simulink model "LabFabSim2022a__2_9_2023_AllAttacks_"  (R2022a)
settings: Solver=VariableStepAuto  StartTime=0.0  StopTime=5500000  RelTol=1e-3  EnableMultiTasking=on
model workspace (MAT data in the model file):
  JsonData : timetable (value not decoded)
  M : Simulink.Parameter (value not decoded)
  ROS_trigger = 0
  SL_ROS_VariableLengthArrays_MaxSizes : object (value not decoded)
undefined symbols (not defined in the file): DOS, DOSinitGen, DTP, DTPGen, DTPInitGen, EmptyLocFound, InitCobot, InitCobotReturn, InitializeSLD, InitLEGO, InitVGRproc2, m, MC, MCGen, MCInitGen, MO, MOGen, MOInitGen, n, NetScan, NetScanInitGen, Spying, SpyingInitGen, WS, WSGen, WSInitGen
libraries: sldelib x6
(part 2 of 4)

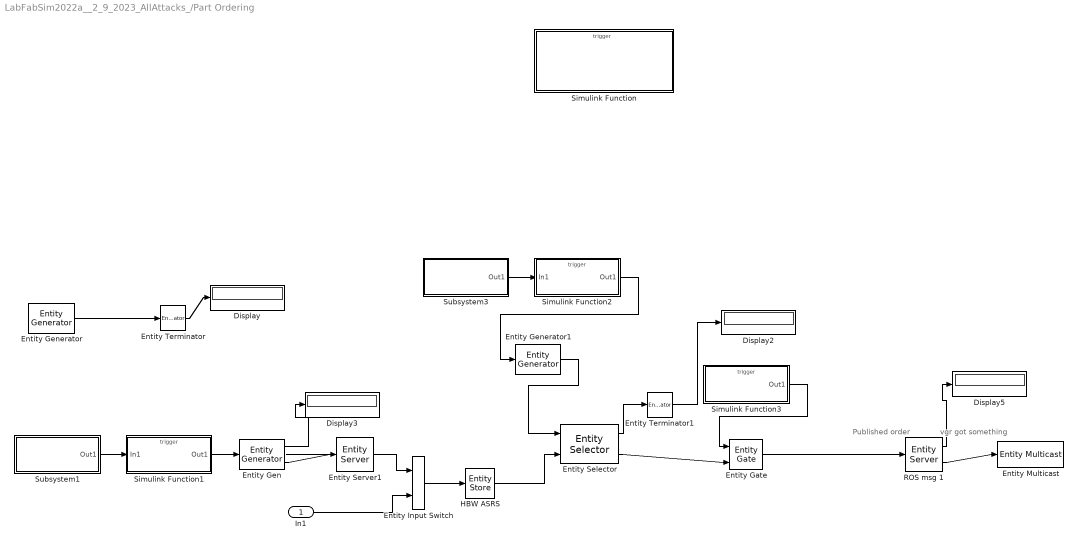
== system LabFabSim2022a__2_9_2023_AllAttacks_/Part Ordering ==
  note: vgr got something
  note: Published order
  In1 : Inport
  Display{,2..3,5} (4 alike) : Display
  Entity Input Switch : EntityInputSwitch  InputPortMessageModes=m,m  OutputPortMessageModes=m
  Entity Gate : EntityGate  InputPortMessageModes=m,m  OutputPortMessageModes=m  OperatingMode=Release gate  OpenGateAtSimulationStart=on
  "Entity Gen " : EntityGenerator  InputPortMessageModes=m  OutputPortMessageModes=n,m  GenerationMethod=Event-based  GenerateAction=|  AttributeName=PartID|ColorID|ServiceProcess|CurrentStep|CurrentRoute|HBW_ServiceTime|LEGO_ServiceTime|SLD_ServiceTime|HBW_Loc|TimeStampGen|TimeStampEnd|TimeStampStart|TotalTimeInSys|EntityRoutedTime|HBWstart_Time|VGRproc1_Time|MPS_Time|SLD_Time|VGRproc2_Time|Cobot2LEGO_Time|LEGO2Cobot_Time|VGRproc3_Time|HBWin_Time  AttributeInitialValue=1|1|zeros(1,11)|0|1|zeros(1)|zeros(1)|zeros(1)|zeros(1)|0|0|0|0|0|0|0|0|0|0|0|0|0|0  NumberEntitiesDeparted=on  EntityType=Structured  EntityTypeName=PartOrder
      | persistent next_id
      | if isempty(next_id)
      |     next_id = 1;
      |     %set seed for random number generation
      |     rng(12345);
      | end
      | 
      | %Assign ID attribute 
      | if next_id <= 9
      |     entity.PartID = next_id;
      |     next_id = next_id + 1
      | end
      | 
      | %Current Step Attribute Setup
      | persistent SEQId;
      | persistent idx2;
      | if isempty(SEQId)
      |     SEQId = 1:15;
      |     idx2 = 1;
      | end
      | if idx2 > numel(SEQId)
      |     idx2 = 1;
      |     entity.PartID = SEQId(idx2);
      | else
      |     entity.PartID = SEQId(idx2);
      | end
      | idx2 = idx2 + 1;
      | entity.CurrentStep=1;
      | 
      | %Randomly Set Order Color 
      | entity.HBW_Loc = randi(3)
      | switch(entity.HBW_Loc)
      |     case 1 
      |         entity.ColorID = 1;
      |         %entity.Color = "red";
      |         %red part ordered
      |     case 2
      |         entity.ColorID = 2;
      |         %entity.Color = "blue";
      |         %blue part ordered 
      |     case 3 
      |         entity.ColorID = 3;
      |         %entity.Color = "white";
      |         %white part ordered 
      | end
      | 
      | %Entity attribute based on color ID
      | if entity.ColorID == 1
      |     entity.ServiceProcess = [2 3 4 5 6 7 8 9 10 11 1];
      |     entity.HBW_ServiceTime = [5];
      |     entity.LEGO_ServiceTime = [4];
      |     entity.SLD_ServiceTime = [6];
      |     
      | else if entity.ColorID == 2
      |     entity.ServiceProcess = [2 3 4 5 6 7 8 9 10 11 1];
      |     entity.HBW_ServiceTime = [6];
      |     entity.LEGO_ServiceTime = [4];
      |     entity.SLD_ServiceTime = [7];
      |     
      | else if entity.ColorID == 3
      |     entity.ServiceProcess = [2 3 4 5 6 7 8 9 10 11 1];
      |     entity.HBW_ServiceTime = [5];
      |     entity.LEGO_ServiceTime = [6];
      |     entity.SLD_ServiceTime = [5];
      | end
      | end
      settings: InputPortMap=u0  OutputPortMap=o0,o3
  Entity Generator : EntityGenerator  OutputPortMessageModes=m  Period=inf  AttributeName=data  EntityType=Structured  EntityTypeName=InitOrders
  Entity Generator1 : EntityGenerator  InputPortMessageModes=m  OutputPortMessageModes=m  GenerationMethod=Event-based  GenerateAction=entity.PartID = randi(9);  AttributeName=PartID  AttributeInitialValue=zeros(1)  EntityType=Structured  EntityTypeName=Order
      settings: InputPortMap=u0
  Entity Multicast : EntityMulticast  Tag=Order  InputPortMessageModes=m  MulticastTag=Order
  Entity Selector : sldelib/Entity Selector  mNumberOfStreams=1  mKeyEntityAttributeName={'PartID'}  mEntityAttributeName={'PartID'}  mMatchingNumberSource=Dialog  mNumberOfMatches=1  mNumberOfMatchesAttribute=Name  mNumEntitiesDepOpt=off  mNumEntitiesInBlockOpt=off  mNumEntitiesExtractedOpt=off
      settings: SourceProductBaseCode=SE
  Entity Server1 : EntityServer  InputPortMessageModes=m  OutputPortMessageModes=m  Capacity=1  ServiceTimeValue=0  EntryAction=entity.TimeStampGen = TimeStamp();
  Entity Terminator : EntityTerminator  InputPortMessageModes=m  EntryAction=|  NumberEntitiesArrived=on
      | EntityGen();
      | EntityGen();
      | EntityGen();
      | EntityGen();
      | EntityGen();
      | EntityGen();
      | EntityGen();
      | EntityGen();
      | EntityGen();
      | 
      | %Initially set attack Routers to closed state
      | DOS_Router(2);
      | NetScan_Router(2);
      | Spying_Router(2);
      | DTP_Router(2);
      | MO_Router(2);
      | WS_Router(2);
      | MC_Router(2);
      | 
      | 
      | % coder.extrinsic("disp");
      | 
      | % a = [1, 1; 
      | %     2, 1; 
      | %     3, 1; 
      | %     4, 1; 
      | %     5, 1; 
      | %     6, 1; 
      | %     7, 1; 
      | %     8, 1; 
      | %     9, 1];
      | % b = [datetime('now'); datetime('now'); datetime('now'); datetime('now'); datetime('now'); datetime('now'); datetime('now'); datetime('now'); datetime('now')];
      | % JsonDataSTART= array2timetable(a, 'VariableNames', {'PartID', 'State'}, 'RowTimes', b);
      | % disp(JsonDataSTART)
      settings: OutputPortMap=o0
  Entity Terminator1 : EntityTerminator  InputPortMessageModes=m  NumberEntitiesArrived=on
      settings: OutputPortMap=o0
  HBW ASRS : EntityStore  InputPortMessageModes=m  OutputPortMessageModes=m  Capacity=9  EntryAction=|  ExitAction=|
      EntryAction=|
      | OrderGen();
      | 
      | % % coder.extrinsic("disp");
      | % % 
      | % % 
      | % %%% JSON UPDATE on part entry %%
      | % % if entity.PartID == 1
      | % %     JsonData.PartID(1) = 1;
      | % %     JsonData.Time(1) = datetime('now');
      | % %     
      | % % elseif entity.PartID == 2
      | % %     JsonData.PartID(2) = 2;
      | % %     JsonData.Time(2) = datetime('now');
      | % %     
      | % % elseif entity.PartID == 3
      | % %     JsonData.PartID(3) = 3;
      | % %     JsonData.Time(3) = datetime('now');
      | % %     
      | % % elseif entity.PartID == 4
      | % %     JsonData.PartID(4) = 4;
      | % %     JsonData.Time(4) = datetime('now');
      | % %     
      | % % elseif entity.PartID == 5
      | % %     JsonData.PartID(5) = 5;
      | % %     JsonData.Time(5) = datetime('now');
      | % %     
      | % % elseif entity.PartID == 6
      | % %     JsonData.PartID(6) = 6;
      | % %     JsonData.Time(6) = datetime('now');
      | % %     
      | % % elseif entity.PartID == 7
      | % %     JsonData.PartID(7) = 7;
      | % %     JsonData.Time(7) = datetime('now');
      | % %     
      | % % elseif entity.PartID == 8
      | % %     JsonData.PartID(8) = 8;
      | % %     JsonData.Time(8) = datetime('now');
      | % %     
      | % % elseif entity.PartID == 9
      | % %     JsonData.PartID(9) = 9;
      | % %     JsonData.Time(9) = datetime('now');
      | % % end
      | % % 
      | % % disp(JsonData)
      ExitAction=|
      | % % % %UpdateArrayOUT();
      | % coder.extrinsic("disp");
      | % a = [1, 1; 2, 1; 3, 1; 4, 1; 5, 1; 6, 1; 7, 1; 8, 1; 9, 1];
      | % % b = [datetime('now')];
      | % 
      | % %% JSON UPDATE on part exit %%
      | % if entity.PartID == 1
      | %     a(1,2) = 0;
      | %     %b(1) = datetime('now');
      | %     %disp(a)
      | %     
      | % elseif entity.PartID == 2
      | %     a(2,2) = 0;
      | %     %b(2) = datetime('now');
      | %     %disp(a)
      | %     
      | % elseif entity.PartID == 3
      | %     a(3,2) = 0;
      | %     %b(3) = datetime('now');
      | %     %disp(a)
      | %     
      | % elseif entity.PartID == 4
      | %     a(4,2) = 0;
      | %     %b(4) = datetime('now');
      | %     %disp(a)
      | %     
      | % elseif entity.PartID == 5
      | %     a(5,2) = 0;
      | %     %b(5) = datetime('now');
      | %     %disp(a)
      | %     
      | % elseif entity.PartID == 6
      | %     a(6,2) = 0;
      | %     %b(6) = datetime('now');
      | %     %disp(a)
      | %     
      | % elseif entity.PartID == 7
      | %     a(7,2) = 0;
      | %     %b(7) = datetime('now');
      | %     %disp(a)
      | %     
      | % elseif entity.PartID == 8
      | %     a(8,2) = 0;
      | %     %b(8) = datetime('now');
      | %     %disp(a)
      | %     
      | % elseif entity.PartID == 9
      | %     a(9,2) = 0;
      | %     %b(9) = datetime('now');
      | %     %disp(a)
      | % end
      | % 
      | % disp('____')
      | % JsonDataUPDATE= array2table(a, 'VariableNames', {'PartID', 'State'});
      | % disp(JsonDataUPDATE)
      settings: OutputPortMap=o4
  ROS msg 1 : EntityServer  InputPortMessageModes=m  OutputPortMessageModes=n,m  Capacity=1  ServiceTimeValue=0.07  EntryAction=|  ExitAction=|  NumberEntitiesDeparted=on
      EntryAction=|
      | entity.TimeStampStart = TimeStamp();
      | 
      | sourceID(3); %main
      | sourceAddress(6); %/order
      | sourceType(4); %order
      | sourceLocation(3); %SCADA system
      | destinationServiceAddress(1); %/hbw_node
      | destinationServiceType(4); %order
      | destinationServiceLocation(1); %Fischertechnik
      | accessedNodeAddress(7); 
      | accessedNodeType(1); %String
      | operation(3); %notify-callback
      | value(41); %Published order
      | Normality(1); %normal
      ExitAction=|
      | sourceID(3); %main
      | sourceAddress(6); %/order
      | sourceType(4); %order
      | sourceLocation(3); %SCADA system
      | destinationServiceAddress(2); %/vgr_node
      | destinationServiceType(4); %order
      | destinationServiceLocation(1); %Fischertechnik
      | accessedNodeAddress(3); 
      | accessedNodeType(1); %String
      | operation(3); %notify-callback
      | value(28); %Published order
      | Normality(1); %normal
      settings: OutputPortMap=o0,o9
  Simulink Function : Subsystem  TreatAsAtomicUnit=on
  Simulink Function1 : Subsystem  TreatAsAtomicUnit=on
  Simulink Function2 : Subsystem  TreatAsAtomicUnit=on
  Simulink Function3 : Subsystem  TreatAsAtomicUnit=on
  Subsystem1 : Subsystem
  Subsystem3 : Subsystem
  wires:
  Entity Terminator/1 -> Display/1
  Subsystem1/1(Out1) -> Simulink Function1/1(In1)
  Simulink Function1/1(Out1) -> "Entity Gen "/1
  HBW ASRS/1 -> Entity Selector/2
  Simulink Function3/1(Out1) -> Entity Gate/1
  ROS msg 1/2 -> Entity Multicast/1
  ROS msg 1/1 -> Display5/1
  "Entity Gen "/1 -> Display3/1
  "Entity Gen "/2 -> Entity Server1/1
  In1/1 -> Entity Input Switch/2
  Entity Selector/1 -> Entity Terminator1/1
  Entity Generator1/1 -> Entity Selector/1
  Subsystem3/1(Out1) -> Simulink Function2/1(In1)
  Simulink Function2/1(Out1) -> Entity Generator1/1
  Entity Terminator1/1 -> Display2/1
  Entity Generator/1 -> Entity Terminator/1
  Entity Input Switch/1 -> HBW ASRS/1
  Entity Server1/1 -> Entity Input Switch/1
  Entity Selector/2 -> Entity Gate/2
  Entity Gate/1 -> ROS msg 1/1

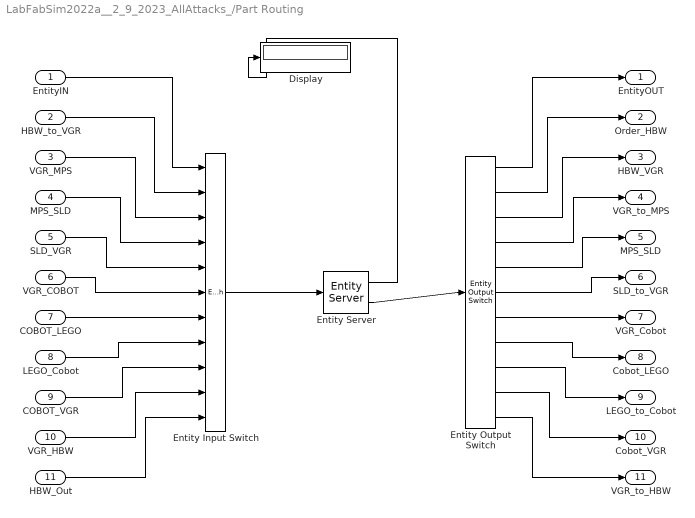
== system LabFabSim2022a__2_9_2023_AllAttacks_/Part Routing ==
  EntityIN : Inport
  HBW_to_VGR : Inport  Port=2
  VGR_MPS : Inport  Port=3
  MPS_SLD : Inport  Port=4
  SLD_VGR : Inport  Port=5
  VGR_COBOT : Inport  Port=6
  COBOT_LEGO : Inport  Port=7
  LEGO_Cobot : Inport  Port=8
  COBOT_VGR : Inport  Port=9
  VGR_HBW : Inport  Port=10
  HBW_Out : Inport  Port=11
  Display : Display
  Entity Input Switch : EntityInputSwitch  InputPortMessageModes=m,m,m,m,m,m,m,m,m,m,m  OutputPortMessageModes=m  NumberInputPorts=11
      settings: InputPortMap=u1,u2,u3,u4,u5,u6,u7,u8,u9,u10,u11
  Entity Output Switch : EntityOutputSwitch  InputPortMessageModes=m  OutputPortMessageModes=m,m,m,m,m,m,m,m,m,m,m  NumberOutputPorts=11  SwitchingCriterion=From attribute  SwitchAttributeName=CurrentRoute
      settings: OutputPortMap=o0,o1,o2,o3,o4,o5,o6,o7,o8,o9,o10
  Entity Server : EntityServer  InputPortMessageModes=m  OutputPortMessageModes=n,m  Capacity=1  ServiceTimeValue=0  EntryAction=|  NumberEntitiesDeparted=on
      | entity.CurrentRoute = entity.ServiceProcess(entity.CurrentStep);
      | entity.CurrentStep = entity.CurrentStep + 1;
      | entity.EntityRoutedTime = TimeStamp();
      settings: OutputPortMap=o0,o9
  EntityOUT : Outport
  Order_HBW : Outport  Port=2
  "HBW_VGR " : Outport  Port=3
  VGR_to_MPS : Outport  Port=4
  "MPS_SLD " : Outport  Port=5
  SLD_to_VGR : Outport  Port=6
  VGR_Cobot : Outport  Port=7
  Cobot_LEGO : Outport  Port=8
  LEGO_to_Cobot : Outport  Port=9
  Cobot_VGR : Outport  Port=10
  VGR_to_HBW : Outport  Port=11
  wires:
  EntityIN/1 -> Entity Input Switch/1
  HBW_to_VGR/1 -> Entity Input Switch/2
  VGR_MPS/1 -> Entity Input Switch/3
  MPS_SLD/1 -> Entity Input Switch/4
  SLD_VGR/1 -> Entity Input Switch/5
  VGR_COBOT/1 -> Entity Input Switch/6
  COBOT_LEGO/1 -> Entity Input Switch/7
  Entity Input Switch/1 -> Entity Server/1
  Entity Server/2 -> Entity Output Switch/1
  Entity Output Switch/1 -> EntityOUT/1
  Entity Output Switch/2 -> Order_HBW/1
  Entity Output Switch/3 -> "HBW_VGR "/1
  Entity Output Switch/4 -> VGR_to_MPS/1
  Entity Output Switch/5 -> "MPS_SLD "/1
  Entity Output Switch/6 -> SLD_to_VGR/1
  Entity Output Switch/7 -> VGR_Cobot/1
  Entity Server/1 -> Display/1
  Entity Output Switch/8 -> Cobot_LEGO/1
  Entity Output Switch/9 -> LEGO_to_Cobot/1
  Entity Output Switch/10 -> Cobot_VGR/1
  Entity Output Switch/11 -> VGR_to_HBW/1
  LEGO_Cobot/1 -> Entity Input Switch/8
  COBOT_VGR/1 -> Entity Input Switch/9
  VGR_HBW/1 -> Entity Input Switch/10
  HBW_Out/1 -> Entity Input Switch/11

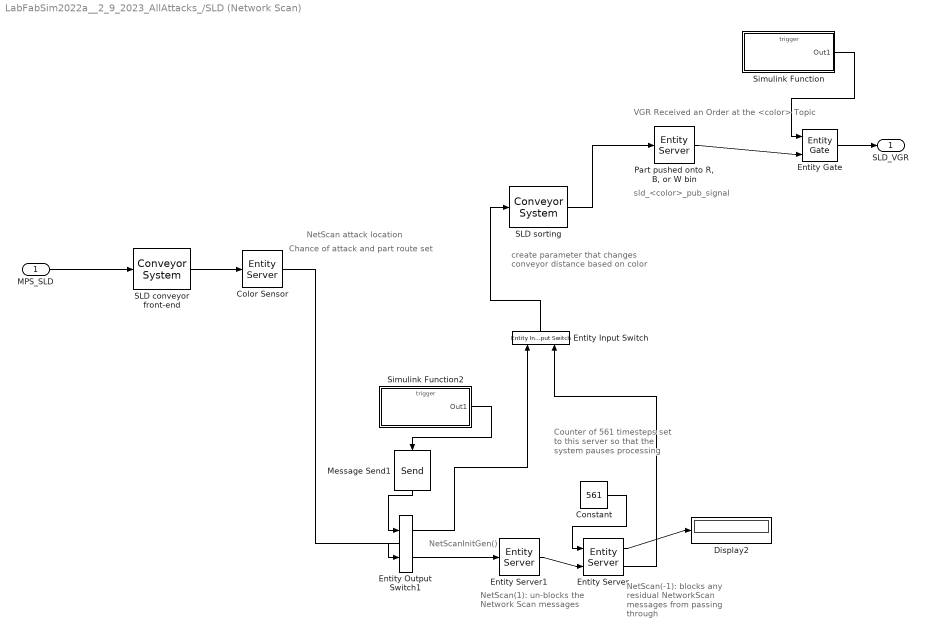
== system LabFabSim2022a__2_9_2023_AllAttacks_/SLD (Network Scan) ==
  note: VGR Received an Order at the <color> Topic
  note: sld_<color>_pub_signal
  note: create parameter that changes
      | conveyor distance based on color
  note: NetScanInitGen()
  note: NetScan(1):
      | un-blocks the Network Scan messages
  note: NetScan(-1):
      | blocks any residual NetworkScan messages from passing through
  note: Counter of 561 timesteps set to this server so that the system pauses processing
  note: Chance of attack and part route set
  note: NetScan attack location
  MPS_SLD : Inport
  Color Sensor : EntityServer  InputPortMessageModes=m  OutputPortMessageModes=m  Capacity=1  ExitAction=|
      | chanceNetScan = rand(1,1)
      | if chanceNetScan < 1.0
      |     %Attack Happening!
      |     NetScan_Router(1);
      | 
      | else
      |     %Normal Behavior
      |     NetScan(-1);
      |     NetScan_Router(2);
      | end
  Constant : Constant  Value=561
  Display2 : Display
  Entity Input Switch : EntityInputSwitch  InputPortMessageModes=m,m  OutputPortMessageModes=m
  Entity Output Switch1 : EntityOutputSwitch  InputPortMessageModes=m,m  OutputPortMessageModes=m,m  SwitchingCriterion=From control port  SwitchAttributeName=Attribute1
      settings: InputPortMap=u0,u1
  Entity Gate : EntityGate  InputPortMessageModes=m,m  OutputPortMessageModes=m  OperatingMode=Release gate
  Entity Server : EntityServer  InputPortMessageModes=n,m  OutputPortMessageModes=n,m  Capacity=1  ServiceTimeSource=Signal port  ExitAction=NetScan(-1);  NumberEntitiesDeparted=on
      settings: InputPortMap=u0,u2  OutputPortMap=o0,o9
  Entity Server1 : EntityServer  InputPortMessageModes=m  OutputPortMessageModes=m  Capacity=1  EntryAction=NetScanInitGen();  ServiceCompleteAction=NetScan(1);
  Message Send1 : Send  OutputPortMessageModes=m
  "Part pushed onto R, B, or W bin" : EntityServer  InputPortMessageModes=m  OutputPortMessageModes=m  Capacity=1  ServiceTimeSource=Attribute  ServiceTimeAttributeName=SLD_ServiceTime  EntryAction=InitVGRproc2();  ExitAction=|
      | sourceID(4); %sld
      | sourceAddress(7); %/vgr_node
      | sourceType(1); %motion sensor
      | sourceLocation(1); %Fischertechnik
      | destinationServiceAddress(2); %/vgr_node
      | destinationServiceType(5); %next task
      | destinationServiceLocation(1); %Fischertechnik
      | accessedNodeAddress(3); 
      | accessedNodeType(2); %String
      | operation(3); %notify-callback
      | Normality(1); %normal
      | 
      | if entity.ColorID == 1
      |     value(19); %VGR Received an Order at the RED Topic
      | else if entity.ColorID == 2
      |     value(18); %VGR Received an Order at the BLUE Topic
      | else    
      |     value(20); %VGR Received an Order at the WHITE Topic
      | end
  SLD conveyor front-end : sldelib/Conveyor System  mConveyorLength=100  mConveyorSpeedSource=Dialog  mConveyorSpeed=1000  mInitialConveyorSpeed=1000  mMinDisBetEntity=0  mEntityLengthSource=Dialog  mEntityLength=1  mEntityLengthAttrName=Length  mOutputBlockedOpt=Accumulate  mErrorUponFullOpt=on  mNumEntitiesDepOpt=off  mNumEntitiesInBlockOpt=off  mEntityPendingOpt=off  mNumExtractedFromBlockOpt=off  mConveyorSpeedOpt=off
      settings: SourceProductBaseCode=SE
  SLD sorting : sldelib/Conveyor System  mConveyorLength=100  mConveyorSpeedSource=Dialog  mConveyorSpeed=1000  mInitialConveyorSpeed=1000  mMinDisBetEntity=0  mEntityLengthSource=Dialog  mEntityLength=1  mEntityLengthAttrName=Length  mOutputBlockedOpt=Accumulate  mErrorUponFullOpt=on  mNumEntitiesDepOpt=off  mNumEntitiesInBlockOpt=off  mEntityPendingOpt=off  mNumExtractedFromBlockOpt=off  mConveyorSpeedOpt=off
      settings: SourceProductBaseCode=SE
  Simulink Function : Subsystem  TreatAsAtomicUnit=on
  Simulink Function2 : Subsystem  TreatAsAtomicUnit=on
  SLD_VGR : Outport
  wires:
  MPS_SLD/1 -> SLD conveyor front-end/1
  SLD conveyor front-end/1 -> Color Sensor/1
  SLD sorting/1 -> "Part pushed onto R, B, or W bin"/1
  "Part pushed onto R, B, or W bin"/1 -> Entity Gate/2
  Entity Gate/1 -> SLD_VGR/1
  Simulink Function/1(Out1) -> Entity Gate/1
  Entity Server/1 -> Display2/1
  Entity Server1/1 -> Entity Server/2
  Entity Server/2 -> Entity Input Switch/2
  Color Sensor/1 -> Entity Output Switch1/2
  Entity Input Switch/1 -> SLD sorting/1
  Constant/1 -> Entity Server/1
  Message Send1/1 -> Entity Output Switch1/1
  Entity Output Switch1/2 -> Entity Server1/1
  Entity Output Switch1/1 -> Entity Input Switch/1
  Simulink Function2/1(Out1) -> Message Send1/1

== system LabFabSim2022a__2_9_2023_AllAttacks_/Spying ==
  note: Source: hbw --> Destination: (2,5)
  note: Entity Gate:
      | set to open when a positive signal value is passed into the control port. Closes when negative.
  note: Recieve signal from Chance-setting Server block for activation signal
  note: Service Time: 50 Timestep
  note: Generates a single entity that causes Spying attack (entity generator) to generate one entity
  note: Sets Spying_id up to 5 and resets to 1 for next Spying attack
  note: On Service Completion: Send a signal to data-logging SimFunctions
  note: Service Time: 110 Timestep
  note: Service Time: 75 Timestep
  note: Service Time: 95 Timestep
  note: Service Time: 150 Timestep
  Display : Display
  Entity Gate : EntityGate  InputPortMessageModes=m,m  OutputPortMessageModes=m
  Entity Generator : EntityGenerator  InputPortMessageModes=m  OutputPortMessageModes=m  GenerationMethod=Event-based  IntergenerationTimeAction=|  GenerateAction=|  AttributeName=Spying_id  EntityType=Structured  EntityTypeName=SpyingAttack
      IntergenerationTimeAction=|
      | chanceDOS = rand(1,1);
      | if chanceDOS < 0.3
      |     dt = 1
      GenerateAction=|
      | persistent next_id_Spying
      | 
      | if isempty(next_id_Spying)
      |     next_id_Spying = 1;
      |     %set seed for random number generation
      |     rng(12345);
      | end
      | 
      | entity.Spying_id = next_id_Spying
      | next_id_Spying = next_id_Spying + 1
      | 
      | if entity.Spying_id == 5
      |     next_id_Spying = 1
      settings: InputPortMap=u0
  Entity Server : EntityServer  InputPortMessageModes=m  OutputPortMessageModes=m  Capacity=1  ServiceTimeValue=50  ServiceCompleteAction=|
      | sourceID(1); %hbw
      | sourceAddress(1); %/hbw_node
      | sourceType(5); %next_task
      | sourceLocation(1); %Fischertechnik
      | destinationServiceAddress(2); %/vgr_node
      | destinationServiceType(1); %Motion Sensor
      | destinationServiceLocation(1); %Fischertechnik
      | accessedNodeAddress(3); 
      | accessedNodeType(2); %Boolean
      | operation(1); %read
      | value(44); %False
      | Normality(6); %anomalous(spying)
  Entity Server1 : EntityServer  InputPortMessageModes=m  OutputPortMessageModes=m  Capacity=1  ServiceTimeValue=110  ServiceCompleteAction=|
      | sourceID(1); %hbw
      | sourceAddress(1); %/hbw_node
      | sourceType(5); %next_task
      | sourceLocation(1); %Fischertechnik
      | destinationServiceAddress(5); %/lego_node
      | destinationServiceType(1); %Motion Sensor
      | destinationServiceLocation(2); %Expansion
      | accessedNodeAddress(5); 
      | accessedNodeType(2); %Boolean
      | operation(1); %read
      | value(44); %False
      | Normality(6); %anomalous(spying)
  Entity Server2 : EntityServer  InputPortMessageModes=m  OutputPortMessageModes=m  Capacity=1  ServiceTimeValue=75  ServiceCompleteAction=|
      | sourceID(1); %hbw
      | sourceAddress(1); %/hbw_node
      | sourceType(5); %next_task
      | sourceLocation(1); %Fischertechnik
      | destinationServiceAddress(2); %/vgr_node
      | destinationServiceType(1); %Motion Sensor
      | destinationServiceLocation(1); %Fischertechnik
      | accessedNodeAddress(3); 
      | accessedNodeType(2); %Boolean
      | operation(1); %read
      | value(44); %False
      | Normality(6); %anomalous(spying)
  Entity Server3 : EntityServer  InputPortMessageModes=m  OutputPortMessageModes=m  Capacity=1  ServiceTimeValue=95  ServiceCompleteAction=|
      | sourceID(1); %hbw
      | sourceAddress(1); %/hbw_node
      | sourceType(5); %next_task
      | sourceLocation(1); %Fischertechnik
      | destinationServiceAddress(5); %/lego_node
      | destinationServiceType(1); %Motion Sensor
      | destinationServiceLocation(2); %Expansion
      | accessedNodeAddress(5);  
      | accessedNodeType(2); %Boolean
      | operation(1); %read
      | value(44); %False
      | Normality(6); %anomalous(spying)
  Entity Server4 : EntityServer  InputPortMessageModes=m  OutputPortMessageModes=m  Capacity=1  ServiceTimeValue=150  ServiceCompleteAction=|
      | sourceID(1); %hbw
      | sourceAddress(1); %/hbw_node
      | sourceType(5); %next_task
      | sourceLocation(1); %Fischertechnik
      | destinationServiceAddress(5); %/lego_node
      | destinationServiceType(1); %Motion Sensor
      | destinationServiceLocation(2); %Expansion
      | accessedNodeAddress(5);  
      | accessedNodeType(2); %Boolean
      | operation(1); %read
      | value(44); %False
      | Normality(6); %anomalous(spying)
  Entity Store : EntityStore  InputPortMessageModes=m  OutputPortMessageModes=m  Capacity=6
      settings: OutputPortMap=o4
  Entity Terminator1 : EntityTerminator  InputPortMessageModes=m  NumberEntitiesArrived=on
      settings: OutputPortMap=o0
  InitSpying : Subsystem
  "Number of Entities Generated from main " : Display
  Simulink Function1 : Subsystem  TreatAsAtomicUnit=on
  Spying : Subsystem  TreatAsAtomicUnit=on
  Subsystem1 : Subsystem
  wires:
  Simulink Function1/1(Out1) -> Entity Generator/1
  Entity Terminator1/1 -> Display/1
  Entity Generator/1 -> Entity Store/1
  Entity Store/1 -> Entity Gate/2
  Entity Server/1 -> Entity Server1/1
  Spying/1(Out1) -> Entity Gate/1
  Subsystem1/1(Out1) -> Simulink Function1/1(In1)
  InitSpying/1(Out1) -> "Number of Entities Generated from main "/1
  Entity Server1/1 -> Entity Server2/1
  Entity Server2/1 -> Entity Server3/1
  Entity Server3/1 -> Entity Server4/1
  Entity Server4/1 -> Entity Terminator1/1
  Entity Gate/1 -> Entity Server/1

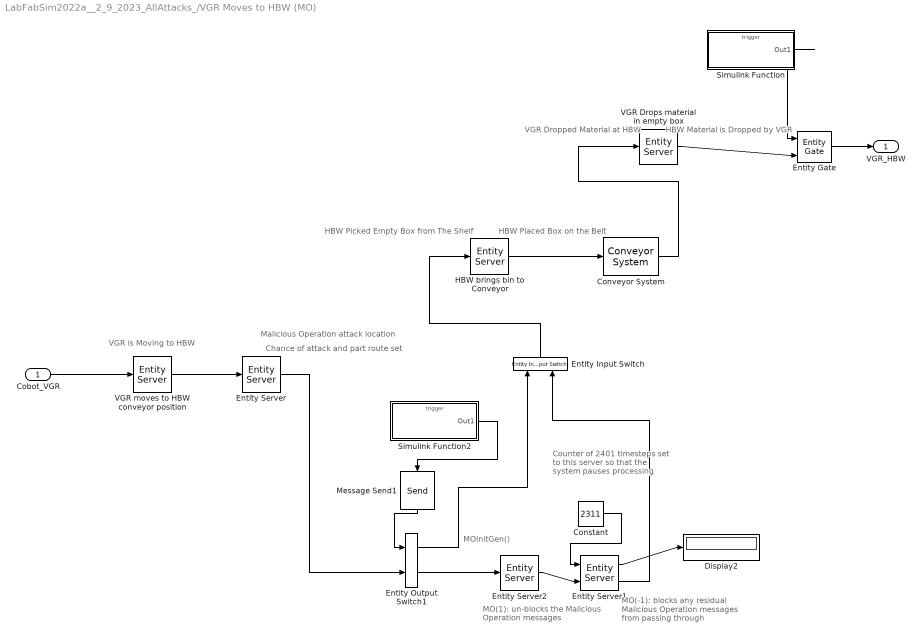
== system LabFabSim2022a__2_9_2023_AllAttacks_/VGR Moves to HBW (MO) ==
  note: HBW Material is Dropped by VGR
  note: VGR Dropped Material at HBW
  note: HBW Placed Box on the Belt
  note: HBW Picked Empty Box from The Shelf
  note: VGR is Moving to HBW
  note: MOInitGen()
  note: MO(-1):
      | blocks any residual Malicious Operation messages from passing through
  note: MO(1):
      | un-blocks the Malicious Operation messages
  note: Counter of 2401 timesteps set to this server so that the system pauses processing
  note: Malicious Operation attack location
  note: Chance of attack and part route set
  Cobot_VGR : Inport
  Constant : Constant  Value=2311
  Conveyor System : sldelib/Conveyor System  mConveyorLength=10  mConveyorSpeedSource=Dialog  mConveyorSpeed=1000  mInitialConveyorSpeed=1000  mMinDisBetEntity=0  mEntityLengthSource=Dialog  mEntityLength=1  mEntityLengthAttrName=Length  mOutputBlockedOpt=Accumulate  mErrorUponFullOpt=on  mNumEntitiesDepOpt=off  mNumEntitiesInBlockOpt=off  mEntityPendingOpt=off  mNumExtractedFromBlockOpt=off  mConveyorSpeedOpt=off
      settings: SourceProductBaseCode=SE
  Display2 : Display
  Entity Input Switch : EntityInputSwitch  InputPortMessageModes=m,m  OutputPortMessageModes=m
  Entity Output Switch1 : EntityOutputSwitch  InputPortMessageModes=m,m  OutputPortMessageModes=m,m  SwitchingCriterion=From control port  SwitchAttributeName=Attribute1
      settings: InputPortMap=u0,u1
  Entity Gate : EntityGate  InputPortMessageModes=m,m  OutputPortMessageModes=m  OperatingMode=Release gate
  Entity Server : EntityServer  InputPortMessageModes=m  OutputPortMessageModes=m  Capacity=1  ServiceTimeValue=9  ExitAction=|
      | chanceMO = rand(1,1)
      | if chanceMO < 0.0
      |     %Attack Happening!
      |     MO_Router(1);
      | 
      | else
      |     %Normal Behavior
      |     MO(-1);
      |     MO_Router(2);
      | end
  Entity Server1 : EntityServer  InputPortMessageModes=n,m  OutputPortMessageModes=n,m  Capacity=1  ServiceTimeSource=Signal port  ExitAction=MO(-1);  NumberEntitiesDeparted=on
      settings: InputPortMap=u0,u2  OutputPortMap=o0,o9
  Entity Server2 : EntityServer  InputPortMessageModes=m  OutputPortMessageModes=m  Capacity=1  EntryAction=MOInitGen();  ServiceCompleteAction=MO(1);
  HBW brings bin to Conveyor : EntityServer  InputPortMessageModes=m  OutputPortMessageModes=m  Capacity=1  ServiceTimeSource=Attribute  ServiceTimeValue=3  ServiceTimeAttributeName=HBW_ServiceTime  EntryAction=|  ExitAction=|
      EntryAction=|
      | sourceID(1); %hbw
      | sourceAddress(1); %/hbw_node
      | sourceType(3); %reference switch
      | sourceLocation(1); %Fischertechnik
      | destinationServiceAddress(1); %/hbw_node
      | destinationServiceType(5); %next task
      | destinationServiceLocation(1); %Fischertechnik
      | accessedNodeAddress(1); 
      | accessedNodeType(1); %String
      | operation(3); %notify-callback
      | value(4); %HBW Picked Empty Box from The Shelf
      | Normality(1); %normal
      ExitAction=|
      | sourceID(1); %hbw
      | sourceAddress(1); %/hbw_node
      | sourceType(1); %Motion Sensor
      | sourceLocation(1); %Fischertechnik
      | destinationServiceAddress(1); %/hbw_node
      | destinationServiceType(5); %next task
      | destinationServiceLocation(1); %Fischertechnik
      | accessedNodeAddress(1); 
      | accessedNodeType(1); %String
      | operation(3); %notify-callback
      | value(6); %HBW Placed Box on the Belt
      | Normality(1); %normal
  Message Send1 : Send  OutputPortMessageModes=m
  Simulink Function : Subsystem  TreatAsAtomicUnit=on
  Simulink Function2 : Subsystem  TreatAsAtomicUnit=on
  VGR Drops material in empty box : EntityServer  InputPortMessageModes=m  OutputPortMessageModes=m  Capacity=1  ServiceTimeValue=6  ServiceTimeAttributeName=HBW_ServiceTime  EntryAction=|  ExitAction=|
      EntryAction=|
      | BinSupplied();
      | 
      | sourceID(1); %hbw
      | sourceAddress(1); %/hbw_node
      | sourceType(1); %Motion Sensor 
      | sourceLocation(1); %Fischertechnik
      | destinationServiceAddress(2); %/vgr_node
      | destinationServiceType(5); %next task
      | destinationServiceLocation(1); %Fischertechnik
      | accessedNodeAddress(3); 
      | accessedNodeType(2); %Boolean
      | operation(3); %notify-callback
      | value(21); %VGR Dropped Material at HBW
      | Normality(1); %normal
      ExitAction=|
      | sourceID(1); %hbw
      | sourceAddress(1); %/hbw_node
      | sourceType(5); %next task
      | sourceLocation(1); %Fischertechnik
      | destinationServiceAddress(1); %/hbw_node
      | destinationServiceType(5); %next task
      | destinationServiceLocation(1); %Fischertechnik
      | accessedNodeAddress(1); 
      | accessedNodeType(1); %String
      | operation(3); %notify-callback
      | value(8); %HBW Material is Dropped by VGR
      | Normality(1); %normal
  VGR moves to HBW conveyor position : EntityServer  InputPortMessageModes=m  OutputPortMessageModes=m  Capacity=1  ServiceTimeValue=3  ServiceCompleteAction=|
      | sourceID(3); %main
      | sourceAddress(6); %/order
      | sourceType(5); %next task
      | sourceLocation(1); %Fischer
      | destinationServiceAddress(2); %/vgr_node
      | destinationServiceType(5); %next task
      | destinationServiceLocation(1); %Fischertechnik
      | accessedNodeAddress(3); 
      | accessedNodeType(1); %String
      | operation(3); %notify-callback
      | value(29); %vgr is moving to hbw
      | Normality(1); %normal
  VGR_HBW : Outport
  wires:
  VGR moves to HBW conveyor position/1 -> Entity Server/1
  Cobot_VGR/1 -> VGR moves to HBW conveyor position/1
  Entity Gate/1 -> VGR_HBW/1
  Simulink Function/1(Out1) -> Entity Gate/1
  HBW brings bin to Conveyor/1 -> Conveyor System/1
  VGR Drops material in empty box/1 -> Entity Gate/2
  Conveyor System/1 -> VGR Drops material in empty box/1
  Entity Server1/1 -> Display2/1
  Constant/1 -> Entity Server1/1
  Entity Input Switch/1 -> HBW brings bin to Conveyor/1
  Entity Server/1 -> Entity Output Switch1/2
  Entity Output Switch1/2 -> Entity Server2/1
  Simulink Function2/1(Out1) -> Message Send1/1
  Entity Server2/1 -> Entity Server1/2
  Entity Server1/2 -> Entity Input Switch/2
  Message Send1/1 -> Entity Output Switch1/1
  Entity Output Switch1/1 -> Entity Input Switch/1

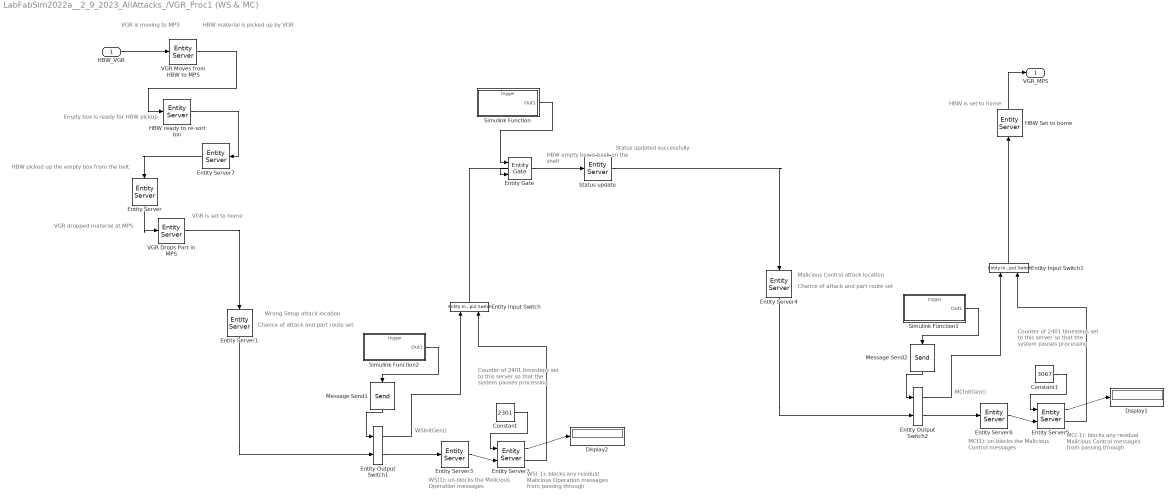
== system LabFabSim2022a__2_9_2023_AllAttacks_/VGR_Proc1 (WS & MC) ==
  note: Status updated successfully
  note: HBW empty box is back on the shelf
  note: HBW is set to home
  note: VGR is set to home
  note: VGR dropped material at MPS
  note: HBW picked up the empty box from the belt
  note: Empty box is ready for HBW pickup
  note: HBW material is picked up by VGR
  note: VGR is moving to MPS
  note: WS(-1):
      | blocks any residual Malicious Operation messages from passing through
  note: Counter of 2401 timesteps set to this server so that the system pauses processing
  note: Chance of attack and part route set
  note: WSInitGen()
  note: WS(1):
      | un-blocks the Malicious Operation messages
  note: Wrong Setup attack location
  note: MC(-1):
      | blocks any residual Malicious Control messages from passing through
  note: MCInitGen()
  note: Chance of attack and part route set
  note: Malicious Control attack location
  note: Counter of 2401 timesteps set to this server so that the system pauses processing
  note: MC(1):
      | un-blocks the Malicious Control messages
  HBW_VGR : Inport
  Constant : Constant  Value=2301
  Constant1 : Constant  Value=3067
  Display1 : Display
  Display2 : Display
  Entity Input Switch : EntityInputSwitch  InputPortMessageModes=m,m  OutputPortMessageModes=m
  Entity Input Switch1 : EntityInputSwitch  InputPortMessageModes=m,m  OutputPortMessageModes=m
  Entity Output Switch1 : EntityOutputSwitch  InputPortMessageModes=m,m  OutputPortMessageModes=m,m  SwitchingCriterion=From control port  SwitchAttributeName=Attribute1
      settings: InputPortMap=u0,u1
  Entity Output Switch2 : EntityOutputSwitch  InputPortMessageModes=m,m  OutputPortMessageModes=m,m  SwitchingCriterion=From control port  SwitchAttributeName=Attribute1
      settings: InputPortMap=u0,u1
  Entity Gate : EntityGate  InputPortMessageModes=m,m  OutputPortMessageModes=m  OperatingMode=Release gate
  Entity Server : EntityServer  InputPortMessageModes=m  OutputPortMessageModes=m  Capacity=1  ServiceTimeValue=10.5  EntryAction=|
      | sourceID(1); %hbw
      | sourceAddress(1); %/hbw_node
      | sourceType(5); %next task
      | sourceLocation(1); %Fischertechnik
      | destinationServiceAddress(1); %/hbw_node
      | destinationServiceType(5); %next task
      | destinationServiceLocation(1); %Fischertechnik
      | accessedNodeAddress(1); 
      | accessedNodeType(1); %String
      | operation(3); %notify-callback
      | value(11); %hbw picked up the empty box from the beltt
      | Normality(1); %normal
  Entity Server1 : EntityServer  InputPortMessageModes=m  OutputPortMessageModes=m  Capacity=1  ServiceTimeValue=0.1  ExitAction=|
      | chanceWS = rand(1,1)
      | if chanceWS < 0.0
      |     %Attack Happening!
      |     WS_Router(1);
      | 
      | else
      |     %Normal Behavior
      |     WS(-1);
      |     WS_Router(2);
      | end
  Entity Server2 : EntityServer  InputPortMessageModes=n,m  OutputPortMessageModes=n,m  Capacity=1  ServiceTimeSource=Signal port  ExitAction=WS(-1);  NumberEntitiesDeparted=on
      settings: InputPortMap=u0,u2  OutputPortMap=o0,o9
  Entity Server3 : EntityServer  InputPortMessageModes=m  OutputPortMessageModes=m  Capacity=1  EntryAction=WSInitGen();  ServiceCompleteAction=WS(1);
  Entity Server4 : EntityServer  InputPortMessageModes=m  OutputPortMessageModes=m  Capacity=1  ServiceTimeValue=0.1  ExitAction=|
      | chanceMC = rand(1,1)
      | if chanceMC < 0.0
      |     %Attack Happening!
      |     MC_Router(1);
      | 
      | else
      |     %Normal Behavior
      |     MC(-1);
      |     MC_Router(2);
      | end
  Entity Server5 : EntityServer  InputPortMessageModes=n,m  OutputPortMessageModes=n,m  Capacity=1  ServiceTimeSource=Signal port  ExitAction=MC(-1);  NumberEntitiesDeparted=on
      settings: InputPortMap=u0,u2  OutputPortMap=o0,o9
  Entity Server6 : EntityServer  InputPortMessageModes=m  OutputPortMessageModes=m  Capacity=1  EntryAction=MCInitGen();  ServiceCompleteAction=MC(1);
  Entity Server7 : EntityServer  InputPortMessageModes=m  OutputPortMessageModes=m  Capacity=1  ServiceTimeValue=1.23
  HBW Set to home : EntityServer  InputPortMessageModes=m  OutputPortMessageModes=m  Capacity=1  ServiceTimeValue=14.5  ExitAction=|
      | sourceID(1); %hbw
      | sourceAddress(1); %/hbw_node
      | sourceType(3); %reference switch
      | sourceLocation(1); %Fischertechnik
      | destinationServiceAddress(3); %/status_update
      | destinationServiceType(5); %next task
      | destinationServiceLocation(1); %Fischertechnik
      | accessedNodeAddress(1); 
      | accessedNodeType(1); %String
      | operation(3); %notify-callback
      | value(15); %hbw robot is set to home
      | Normality(1); %normal
  HBW ready to re-sort bin : EntityServer  InputPortMessageModes=m  OutputPortMessageModes=m  Capacity=1  ServiceTimeValue=2  ServiceCompleteAction=|
      | sourceID(1); %hbw
      | sourceAddress(1); %/hbw_node
      | sourceType(1); %Motion Sensor
      | sourceLocation(1); %Fischertechnik
      | destinationServiceAddress(1); %/hbw_node
      | destinationServiceType(5); %next task
      | destinationServiceLocation(1); %Fischertechnik
      | accessedNodeAddress(1); 
      | accessedNodeType(1); %String
      | operation(3); %notify-callback
      | value(9); %Empty box is ready for HBW pickup
      | Normality(1); %normal
  Message Send1 : Send  OutputPortMessageModes=m
  Message Send2 : Send  OutputPortMessageModes=m
  Simulink Function : Subsystem  TreatAsAtomicUnit=on
  Simulink Function1 : Subsystem  TreatAsAtomicUnit=on
  Simulink Function2 : Subsystem  TreatAsAtomicUnit=on
  Status update : EntityServer  InputPortMessageModes=m  OutputPortMessageModes=m  Capacity=1  ServiceTimeValue=0.5  ServiceCompleteAction=|  ExitAction=|
      | sourceID(1); %hbw
      | sourceAddress(1); %/hbw_node
      | sourceType(5); %next task
      | sourceLocation(1); %Fischertechnik
      | destinationServiceAddress(3); %/status_update
      | destinationServiceType(5); %next task
      | destinationServiceLocation(1); %Fischertechnik
      | accessedNodeAddress(1); 
      | accessedNodeType(1); %String
      | operation(3); %notify-callback
      | value(13); %hbw empty box is back on the shelf
      | Normality(1); %normal
      | sourceID(1); %hbw
      | sourceAddress(1); %/hbw_node
      | sourceType(5); %next task
      | sourceLocation(1); %Fischertechnik
      | destinationServiceAddress(3); %/status_update
      | destinationServiceType(5); %next task
      | destinationServiceLocation(1); %Fischertechnik
      | accessedNodeAddress(6); 
      | accessedNodeType(1); %String
      | operation(3); %notify-callback
      | value(42); %Status Updated Successfully
      | Normality(1); %normal
  VGR Drops Part in MPS : EntityServer  InputPortMessageModes=m  OutputPortMessageModes=m  Capacity=1  ServiceTimeValue=15.5  EntryAction=|  ExitAction=|
      EntryAction=|
      | MPS_Initialize();
      | 
      | sourceID(2); %vgr
      | sourceAddress(2); %/vgr_node
      | sourceType(5); %next task
      | sourceLocation(1); %Fischertechnik
      | destinationServiceAddress(2); %/vgr_node
      | destinationServiceType(1); %motion sensor
      | destinationServiceLocation(1); %Fischertechnik
      | accessedNodeAddress(3); 
      | accessedNodeType(1); %String
      | operation(3); %notify-callback
      | value(32); %vgr dropped material at MPS
      | Normality(1); %normal
      ExitAction=|
      | sourceID(2); %vgr
      | sourceAddress(2); %/vgr_node
      | sourceType(5); %next task
      | sourceLocation(1); %Fischertechnik
      | destinationServiceAddress(2); %/vgr_node
      | destinationServiceType(3); %reference switch
      | destinationServiceLocation(1); %Fischertechnik
      | accessedNodeAddress(3); 
      | accessedNodeType(1); %String
      | operation(3); %notify-callback
      | value(16); %vgr is set to home
      | Normality(1); %normal
  VGR Moves from HBW to MPS : EntityServer  InputPortMessageModes=m  OutputPortMessageModes=m  Capacity=1  ServiceTimeValue=1.5  EntryAction=|  ExitAction=|
      EntryAction=|
      | sourceID(2); %vgr
      | sourceAddress(2); %/vgr_node
      | sourceType(3); %reference switch
      | sourceLocation(1); %Fischertechnik
      | destinationServiceAddress(2); %/vgr_node
      | destinationServiceType(5); %next task
      | destinationServiceLocation(1); %Fischertechnik
      | accessedNodeAddress(3); 
      | accessedNodeType(1); %String
      | operation(3); %notify-callback
      | value(31); %VGR is moving to MPS
      | Normality(1); %normal
      ExitAction=|
      | sourceID(1); %hbw
      | sourceAddress(1); %/hbw_node
      | sourceType(5); %next task
      | sourceLocation(1); %Fischertechnik
      | destinationServiceAddress(1); %/hbw_node
      | destinationServiceType(5); %next task
      | destinationServiceLocation(1); %Fischertechnik
      | accessedNodeAddress(1); 
      | accessedNodeType(1); %String
      | operation(3); %notify-callback
      | value(7); %hbw material is picked up by vgr
      | Normality(1); %normal
  VGR_MPS : Outport
  wires:
  Simulink Function/1(Out1) -> Entity Gate/1
  VGR Moves from HBW to MPS/1 -> HBW ready to re-sort bin/1
  HBW ready to re-sort bin/1 -> Entity Server7/1
  HBW_VGR/1 -> VGR Moves from HBW to MPS/1
  VGR Drops Part in MPS/1 -> Entity Server1/1
  Entity Gate/1 -> Status update/1
  HBW Set to home/1 -> VGR_MPS/1
  Entity Server/1 -> VGR Drops Part in MPS/1
  Entity Input Switch/1 -> Entity Gate/2
  Entity Server1/1 -> Entity Output Switch1/2
  Entity Server3/1 -> Entity Server2/2
  Simulink Function2/1(Out1) -> Message Send1/1
  Entity Output Switch1/1 -> Entity Input Switch/1
  Message Send1/1 -> Entity Output Switch1/1
  Entity Server2/2 -> Entity Input Switch/2
  Entity Output Switch1/2 -> Entity Server3/1
  Constant/1 -> Entity Server2/1
  Entity Server2/1 -> Display2/1
  Status update/1 -> Entity Server4/1
  Entity Input Switch1/1 -> HBW Set to home/1
  Entity Server5/1 -> Display1/1
  Entity Server4/1 -> Entity Output Switch2/2
  Entity Output Switch2/2 -> Entity Server6/1
  Message Send2/1 -> Entity Output Switch2/1
  Simulink Function1/1(Out1) -> Message Send2/1
  Entity Server5/2 -> Entity Input Switch1/2
  Entity Output Switch2/1 -> Entity Input Switch1/1
  Constant1/1 -> Entity Server5/1
  Entity Server6/1 -> Entity Server5/2
  Entity Server7/1 -> Entity Server/1

== system LabFabSim2022a__2_9_2023_AllAttacks_/VGR_Proc2 (Spying) ==
  note: vgr is set to home
  note: vgr dropped material at DPS
  note: Spying(1):
      | un-blocks the Spying messages
  note: SpyingInitGen()
  note: Counter of 2401 timesteps set to this server so that the system pauses processing
  note: Spying(-1):
      | blocks any residual Spying messages from passing through
  note: Spying attack location
  note: Chance of attack and part route set
  SLD_VGR : Inport
  Constant : Constant  Value=2401
  Display2 : Display
  Dropped on Cobot pickup loc : EntityServer  InputPortMessageModes=m  OutputPortMessageModes=m  Capacity=1  ServiceTimeValue=1  ServiceTimeAttributeName=HBW_ServiceTime  EntryAction=InitCobot();  ExitAction=|
      | sourceID(2); %vgr
      | sourceAddress(2); %/vgr_node
      | sourceType(5); %next task
      | sourceLocation(1); %Fischertechnik
      | destinationServiceAddress(2); %/vgr_node
      | destinationServiceType(1); %motion sensor
      | destinationServiceLocation(1); %Fischertechnik
      | accessedNodeAddress(3); 
      | accessedNodeType(1); %String
      | operation(3); %notify-callback
      | value(17); %vgr dropped material at DPS
      | Normality(1); %normal
  Entity Input Switch : EntityInputSwitch  InputPortMessageModes=m,m  OutputPortMessageModes=m
  Entity Output Switch1 : EntityOutputSwitch  InputPortMessageModes=m,m  OutputPortMessageModes=m,m  SwitchingCriterion=From control port  SwitchAttributeName=Attribute1
      settings: InputPortMap=u0,u1
  Entity Gate : EntityGate  InputPortMessageModes=m,m  OutputPortMessageModes=m  OperatingMode=Release gate
  Entity Server : EntityServer  InputPortMessageModes=n,m  OutputPortMessageModes=n,m  Capacity=1  ServiceTimeSource=Signal port  ExitAction=Spying(-1);  NumberEntitiesDeparted=on
      settings: InputPortMap=u0,u2  OutputPortMap=o0,o9
  Entity Server1 : EntityServer  InputPortMessageModes=m  OutputPortMessageModes=m  Capacity=1  EntryAction=SpyingInitGen();  ServiceCompleteAction=Spying(1);
  Message Send1 : Send  OutputPortMessageModes=m
  "Move to pickup part from SLD bin " : EntityServer  InputPortMessageModes=m  OutputPortMessageModes=m  Capacity=1  ServiceTimeSource=Attribute  ServiceTimeValue=3  ServiceTimeAttributeName=SLD_ServiceTime  ExitAction=|
      | chanceSpying = rand(1,1)
      | if chanceSpying < 0.0
      |     %Attack Happening!
      |     Spying_Router(1);
      | 
      | else
      |     %Normal Behavior
      |     Spying(-1);
      |     Spying_Router(2);
      | end
  Pump On; Moving to Cobot pickup : EntityServer  InputPortMessageModes=m  OutputPortMessageModes=m  Capacity=1  ServiceTimeSource=Attribute  ServiceTimeValue=3  ServiceTimeAttributeName=SLD_ServiceTime
  Simulink Function : Subsystem  TreatAsAtomicUnit=on
  Simulink Function2 : Subsystem  TreatAsAtomicUnit=on
  VGR sent home : EntityServer  InputPortMessageModes=m  OutputPortMessageModes=m  Capacity=1  ServiceTimeValue=7  ServiceTimeAttributeName=SLD_ServiceTime  ExitAction=|
      | sourceID(2); %vgr
      | sourceAddress(2); %/vgr_node
      | sourceType(5); %next task
      | sourceLocation(1); %Fischertechnik
      | destinationServiceAddress(2); %/vgr_node
      | destinationServiceType(3); %reference switch
      | destinationServiceLocation(1); %Fischertechnik
      | accessedNodeAddress(3); 
      | accessedNodeType(1); %String
      | operation(3); %notify-callback
      | value(16); %vgr is set to home
      | Normality(1); %normal
  VGR_Cobot : Outport
  wires:
  SLD_VGR/1 -> "Move to pickup part from SLD bin "/1
  Pump On; Moving to Cobot pickup/1 -> Dropped on Cobot pickup loc/1
  Dropped on Cobot pickup loc/1 -> VGR sent home/1
  Entity Gate/1 -> VGR_Cobot/1
  Simulink Function/1(Out1) -> Entity Gate/1
  VGR sent home/1 -> Entity Gate/2
  Entity Output Switch1/1 -> Entity Input Switch/1
  Entity Output Switch1/2 -> Entity Server1/1
  Message Send1/1 -> Entity Output Switch1/1
  Simulink Function2/1(Out1) -> Message Send1/1
  Entity Server/2 -> Entity Input Switch/2
  Entity Server1/1 -> Entity Server/2
  "Move to pickup part from SLD bin "/1 -> Entity Output Switch1/2
  Entity Input Switch/1 -> Pump On; Moving to Cobot pickup/1
  Constant/1 -> Entity Server/1
  Entity Server/1 -> Display2/1
